simulink model "PID"  (R2020b)
settings: Solver=VariableStepAuto  StartTime=0.0  StopTime=300.0  RelTol=1e-3
values from neighbouring files (symbols this model uses):
  Kp = (1.2*time_constant)/(gain*(time_delay+sampling_period))-(0.5*Ki)/gain    [Takahashi_PID.m]    (also in ZieglerNichols_PID.m = (1.2*time_constant)/(gain*time_delay))
  T = 0.01    [Zadatak_3.m]
  Td = (Kd*sampling_period)/Kp    [Takahashi_PID.m]    (also in ZieglerNichols_PID.m = 0.5*time_delay)
  Ti = (Kp*sampling_period)/Ki    [Takahashi_PID.m]    (also in ZieglerNichols_PID.m = 2*time_delay)
libraries: simulink x1
settings Model: Creator=user  LastModifiedBy=user

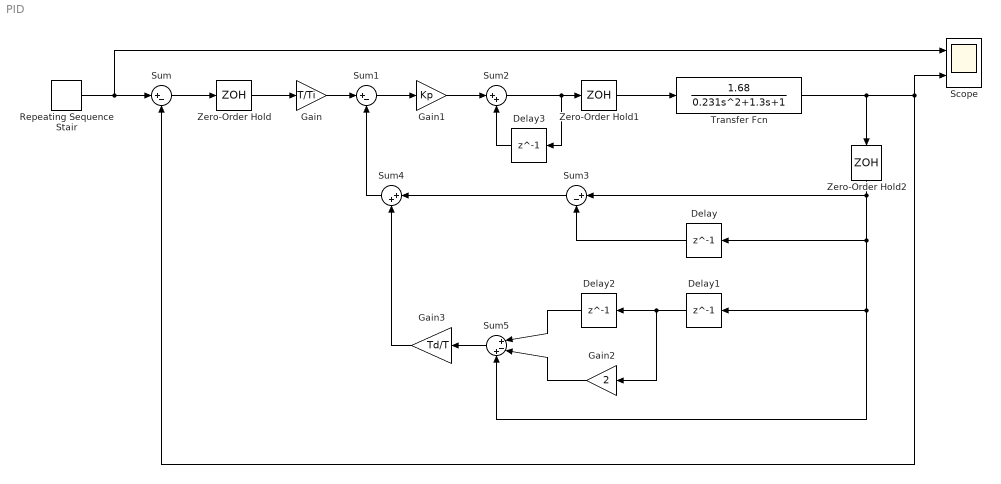
== system PID ==
  Delay{,1..3} (4 alike) : Delay  DelayLength=1
  Gain : Gain  Gain=T/Ti
  Gain1 : Gain  Gain=Kp
  Gain2 : Gain  Gain=2
  Gain3 : Gain  Gain=Td/T
  Repeating Sequence Stair : simulink/Sources/Repeating Sequence Stair  OutValues=[3 1 -5 2 1].'  tsamp=50  OutMin=[]  OutMax=[]  OutDataTypeStr=double  OutputDataTypeScalingMode=double  OutDataType=fixdt(0,8)  ConRadixGroup=Best Precision: Vector-wise  OutScaling=2^-12
  Scope : Scope  NumInputPorts=2
  Sum : Sum  Inputs=|+-
  Sum1 : Sum  Inputs=|+-
  Sum2 : Sum  Inputs=|++
  Sum3 : Sum  Inputs=|+-
  Sum4 : Sum  Inputs=|++
  Sum5 : Sum  Inputs=|+-+
  Transfer Fcn : TransferFcn  Numerator=[1.68]  Denominator=[0.231 1.3 1]
  Zero-Order Hold : ZeroOrderHold  SampleTime=0.01
  Zero-Order Hold1 : ZeroOrderHold  SampleTime=0.01
  Zero-Order Hold2 : ZeroOrderHold  SampleTime=0.01
  wires:
  Delay2/1 -> Sum5/1
  Transfer Fcn/1 -> Sum/2, Scope/2, Zero-Order Hold2/1
  Gain2/1 -> Sum5/2
  Zero-Order Hold/1 -> Gain/1
  Sum/1 -> Zero-Order Hold/1
  Sum2/1 -> Delay3/1, Zero-Order Hold1/1
  Sum1/1 -> Gain1/1
  Sum5/1 -> Gain3/1
  Delay3/1 -> Sum2/2
  Gain/1 -> Sum1/1
  Sum3/1 -> Sum4/1
  Gain3/1 -> Sum4/2
  Sum4/1 -> Sum1/2
  Delay1/1 -> Gain2/1, Delay2/1
  Repeating Sequence Stair/1 -> Scope/1, Sum/1
  Gain1/1 -> Sum2/1
  Zero-Order Hold2/1 -> Sum3/1, Delay/1, Delay1/1, Sum5/3
  Zero-Order Hold1/1 -> Transfer Fcn/1
  Delay/1 -> Sum3/2
